simulink model "ex8_4"  (R2021b)
settings: Solver=VariableStepAuto  StartTime=0.0  StopTime=5  FixedStep=1e-4  EnableMultiTasking=on
settings Model: Creator=user  LastModifiedBy=chesterXalan
settings SolverCC: AlgebraicLoopSolver=TrustRegion
settings DataIOCC: LimitDataPoints=on  ReturnWorkspaceOutputs=off
settings OptimizationCC: LifeSpan=inf
settings DebuggingCC: AllowSymbolicDim=off  SFUnexpectedBacktrackingDiag=warning  SFNoUnconditionalDefaultTransitionDiag=warning  SFExecutionAtInitializationDiag=none  SFMachineParentedDataDiag=warning  ArithmeticOperatorsInVariantConditions=warning
settings ModelReferenceCC: PropagateSignalLabelsOutOfModel=off
settings SFSimCC: SimUseLocalCustomCode=off  CustomCodeUndefinedFunction=UseInterfaceOnly
settings RTWCC: RTWUseLocalCustomCode=off
settings CodeAppCC: StateflowObjectComments=on
settings GRTTargetCC: TargetLangStandard=C89/C90 (ANSI)
settings ConfigComp: CovMetricSettings=dw  CovSaveCumulativeToWorkspaceVar=on  CovSaveSingleToWorkspaceVar=on  CovExternalEMLEnable=off

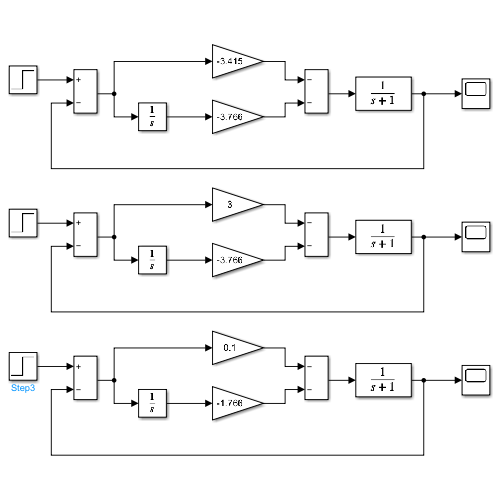
[thumbnail: Simulink's stored preview of the top-level diagram]
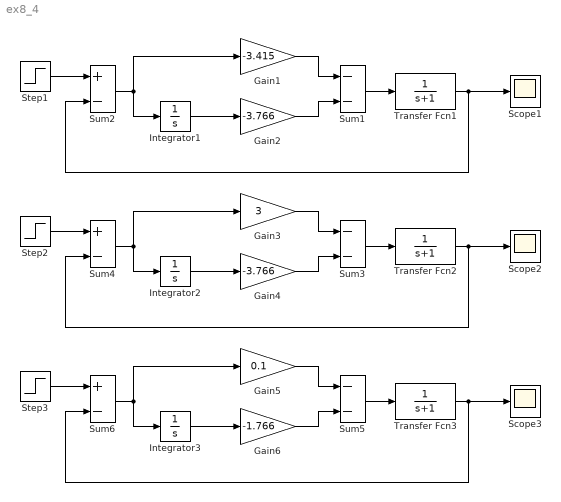
== system ex8_4 ==
  Gain1 : Gain  Gain=-3.415
  Gain2 : Gain  Gain=-3.766
  Gain3 : Gain  Gain=3
  Gain4 : Gain  Gain=-3.766
  Gain5 : Gain  Gain=0.1
  Gain6 : Gain  Gain=-1.766
  Integrator1 : Integrator
  Integrator2 : Integrator
  Integrator3 : Integrator
  Scope1 : Scope
  Scope2 : Scope
  Scope3 : Scope
  Step1 : Step  Time=0.01  SampleTime=1e-3
  Step2 : Step  Time=0.01  SampleTime=1e-3
  Step3 : Step  Time=0.01  SampleTime=1e-3
  Sum1 : Sum  Inputs=--
  Sum2 : Sum  Inputs=+-
  Sum3 : Sum  Inputs=--
  Sum4 : Sum  Inputs=+-
  Sum5 : Sum  Inputs=--
  Sum6 : Sum  Inputs=+-
  Transfer Fcn1 : TransferFcn  Denominator=[1 1]
  Transfer Fcn2 : TransferFcn  Denominator=[1 1]
  Transfer Fcn3 : TransferFcn  Denominator=[1 1]
  wires:
  Step1/1 -> Sum2/1
  Transfer Fcn1/1 -> Scope1/1, Sum2/2
  Sum1/1 -> Transfer Fcn1/1
  Sum2/1 -> Integrator1/1, Gain1/1
  Integrator1/1 -> Gain2/1
  Gain2/1 -> Sum1/2
  Gain1/1 -> Sum1/1
  Step2/1 -> Sum4/1
  Transfer Fcn2/1 -> Scope2/1, Sum4/2
  Sum3/1 -> Transfer Fcn2/1
  Sum4/1 -> Integrator2/1, Gain3/1
  Integrator2/1 -> Gain4/1
  Gain4/1 -> Sum3/2
  Gain3/1 -> Sum3/1
  Step3/1 -> Sum6/1
  Transfer Fcn3/1 -> Scope3/1, Sum6/2
  Sum5/1 -> Transfer Fcn3/1
  Sum6/1 -> Integrator3/1, Gain5/1
  Integrator3/1 -> Gain6/1
  Gain6/1 -> Sum5/2
  Gain5/1 -> Sum5/1
